simulink library "csu_avm_adio_veh_msg_creator_lib"  (R2014b)
settings: Solver=ode45  StartTime=0.0  StopTime=10.0  RelTol=1e-3
libraries: util_info_lib x1, util_common_lib x1
settings Model: Creator=escrane  LastModifiedBy=mstewart

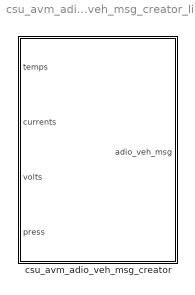
== system csu_avm_adio_veh_msg_creator_lib ==
  csu_avm_adio_veh_msg_creator : Subsystem

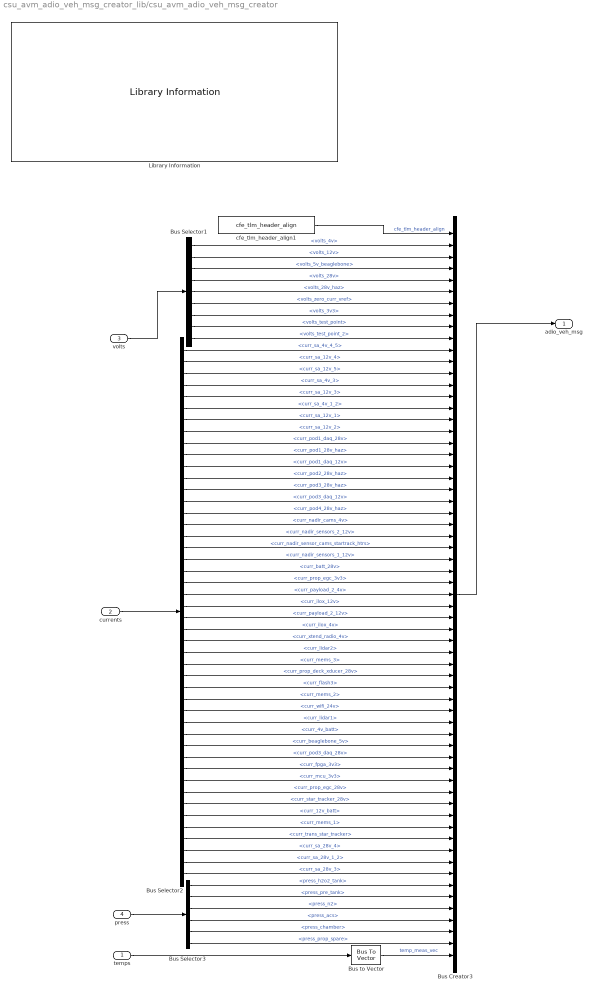
== system csu_avm_adio_veh_msg_creator_lib/csu_avm_adio_veh_msg_creator ==
  temps : Inport
  currents : Inport  Port=2
  volts : Inport  Port=3
  press : Inport  Port=4
  Bus Creator3 : BusCreator  Inputs=63  OutDataTypeStr=Bus: adio_veh_msg  NonVirtualBus=on
  Bus Selector1 : BusSelector  OutputSignals=volts_4v,volts_12v,volts_5v_beaglebone,volts_28v,volts_28v_haz,volts_zero_curr_vref,volts_3v3,volts_test_point,volts_test_point_2
  Bus Selector2 : BusSelector  OutputSignals=curr_sa_4v_4_5,curr_sa_12v_4,curr_sa_12v_5,curr_sa_4v_3,curr_sa_12v_3,curr_sa_4v_1_2,curr_sa_12v_1,curr_sa_12v_2,curr_pod1_daq_28v,curr_pod1_28v_haz,curr_pod1_daq_12v,curr_pod2_28v_haz,curr_pod3_28v_haz,curr_pod3_daq_12v,curr_pod4_28v_haz,curr_nadir_cams_4v,curr_nadir_sensors_2_12v,curr_nadir_sensor_cams_startrack_htrs,curr_nadir_sensors_1_12v,curr_batt_28v,curr_prop_egc_3v3,curr_payload_2_4v,curr_ilox_12v,curr_payload_2_12v,curr_ilox_4v,curr_xtend_radio_4v,curr_lidar2,curr_mems_3,curr_prop_deck_xducer_28v,curr_flash3,curr_mems_2,curr_wifi_24v,curr_lidar1,curr_4v_batt,curr_beaglebone_5v,curr_pod3_daq_28v,curr_fpga_3v3,curr_mcu_3v3,curr_prop_egc_28v,curr_star_tracker_28v,curr_12v_batt,curr_mems_1,curr_trans_star_tracker,curr_sa_28v_4,curr_sa_28v_1_2,curr_sa_28v_3
  Bus Selector3 : BusSelector  OutputSignals=press_h2o2_tank,press_pre_tank,press_n2,press_acs,press_chamber,press_prop_spare
  Bus to Vector : BusToVector
  Library Information : util_info_lib/Library Information  owner='NONE'
  cfe_tlm_header_align1 : util_common_lib/cfe_tlm_header_align
  adio_veh_msg : Outport
  wires:
  cfe_tlm_header_align1/1 -> Bus Creator3/1  "cfe_tlm_header_align"
  Bus Creator3/1 -> adio_veh_msg/1
  Bus to Vector/1 -> Bus Creator3/63  "temp_meas_vec"
  temps/1 -> Bus to Vector/1
  currents/1 -> Bus Selector2/1
  volts/1 -> Bus Selector1/1
  Bus Selector1/3 -> Bus Creator3/4  "<volts_5v_beaglebone>"
  Bus Selector1/8 -> Bus Creator3/9  "<volts_test_point>"
  Bus Selector1/2 -> Bus Creator3/3  "<volts_12v>"
  Bus Selector1/7 -> Bus Creator3/8  "<volts_3v3>"
  Bus Selector1/5 -> Bus Creator3/6  "<volts_28v_haz>"
  Bus Selector1/4 -> Bus Creator3/5  "<volts_28v>"
  Bus Selector1/6 -> Bus Creator3/7  "<volts_zero_curr_vref>"
  Bus Selector1/1 -> Bus Creator3/2  "<volts_4v>"
  Bus Selector1/9 -> Bus Creator3/10  "<volts_test_point_2>"
  press/1 -> Bus Selector3/1
  Bus Selector3/3 -> Bus Creator3/59  "<press_n2>"
  Bus Selector3/2 -> Bus Creator3/58  "<press_pre_tank>"
  Bus Selector3/4 -> Bus Creator3/60  "<press_acs>"
  Bus Selector3/1 -> Bus Creator3/57  "<press_h2o2_tank>"
  Bus Selector3/6 -> Bus Creator3/62  "<press_prop_spare>"
  Bus Selector3/5 -> Bus Creator3/61  "<press_chamber>"
  Bus Selector2/1 -> Bus Creator3/11  "<curr_sa_4v_4_5>"
  Bus Selector2/2 -> Bus Creator3/12  "<curr_sa_12v_4>"
  Bus Selector2/17 -> Bus Creator3/27  "<curr_nadir_sensors_2_12v>"
  Bus Selector2/18 -> Bus Creator3/28  "<curr_nadir_sensor_cams_startrack_htrs>"
  Bus Selector2/19 -> Bus Creator3/29  "<curr_nadir_sensors_1_12v>"
  Bus Selector2/20 -> Bus Creator3/30  "<curr_batt_28v>"
  Bus Selector2/45 -> Bus Creator3/55  "<curr_sa_28v_1_2>"
  Bus Selector2/40 -> Bus Creator3/50  "<curr_star_tracker_28v>"
  Bus Selector2/5 -> Bus Creator3/15  "<curr_sa_12v_3>"
  Bus Selector2/6 -> Bus Creator3/16  "<curr_sa_4v_1_2>"
  Bus Selector2/7 -> Bus Creator3/17  "<curr_sa_12v_1>"
  Bus Selector2/8 -> Bus Creator3/18  "<curr_sa_12v_2>"
  Bus Selector2/3 -> Bus Creator3/13  "<curr_sa_12v_5>"
  Bus Selector2/4 -> Bus Creator3/14  "<curr_sa_4v_3>"
  Bus Selector2/46 -> Bus Creator3/56  "<curr_sa_28v_3>"
  Bus Selector2/33 -> Bus Creator3/43  "<curr_lidar1>"
  Bus Selector2/34 -> Bus Creator3/44  "<curr_4v_batt>"
  Bus Selector2/35 -> Bus Creator3/45  "<curr_beaglebone_5v>"
  Bus Selector2/36 -> Bus Creator3/46  "<curr_pod3_daq_28v>"
  Bus Selector2/9 -> Bus Creator3/19  "<curr_pod1_daq_28v>"
  Bus Selector2/10 -> Bus Creator3/20  "<curr_pod1_28v_haz>"
  Bus Selector2/11 -> Bus Creator3/21  "<curr_pod1_daq_12v>"
  Bus Selector2/12 -> Bus Creator3/22  "<curr_pod2_28v_haz>"
  Bus Selector2/21 -> Bus Creator3/31  "<curr_prop_egc_3v3>"
  Bus Selector2/22 -> Bus Creator3/32  "<curr_payload_2_4v>"
  Bus Selector2/23 -> Bus Creator3/33  "<curr_ilox_12v>"
  Bus Selector2/24 -> Bus Creator3/34  "<curr_payload_2_12v>"
  Bus Selector2/25 -> Bus Creator3/35  "<curr_ilox_4v>"
  Bus Selector2/26 -> Bus Creator3/36  "<curr_xtend_radio_4v>"
  Bus Selector2/27 -> Bus Creator3/37  "<curr_lidar2>"
  Bus Selector2/28 -> Bus Creator3/38  "<curr_mems_3>"
  Bus Selector2/42 -> Bus Creator3/52  "<curr_mems_1>"
  Bus Selector2/41 -> Bus Creator3/51  "<curr_12v_batt>"
  Bus Selector2/39 -> Bus Creator3/49  "<curr_prop_egc_28v>"
  Bus Selector2/29 -> Bus Creator3/39  "<curr_prop_deck_xducer_28v>"
  Bus Selector2/30 -> Bus Creator3/40  "<curr_flash3>"
  Bus Selector2/31 -> Bus Creator3/41  "<curr_mems_2>"
  Bus Selector2/32 -> Bus Creator3/42  "<curr_wifi_24v>"
  Bus Selector2/13 -> Bus Creator3/23  "<curr_pod3_28v_haz>"
  Bus Selector2/14 -> Bus Creator3/24  "<curr_pod3_daq_12v>"
  Bus Selector2/15 -> Bus Creator3/25  "<curr_pod4_28v_haz>"
  Bus Selector2/16 -> Bus Creator3/26  "<curr_nadir_cams_4v>"
  Bus Selector2/44 -> Bus Creator3/54  "<curr_sa_28v_4>"
  Bus Selector2/37 -> Bus Creator3/47  "<curr_fpga_3v3>"
  Bus Selector2/38 -> Bus Creator3/48  "<curr_mcu_3v3>"
  Bus Selector2/43 -> Bus Creator3/53  "<curr_trans_star_tracker>"
